simulink library "My_FI_Operations_ML2017a"  (R2017a)
settings: Solver=VariableStepAuto  StartTime=0.0  StopTime=10.0  RelTol=1e-3
settings Model: Creator=kolbe  LastModifiedBy=kolbe
settings DataIOCC: ReturnWorkspaceOutputs=on
settings SFSimCC: SimUseLocalCustomCode=on
settings RTWCC: RTWUseLocalCustomCode=on

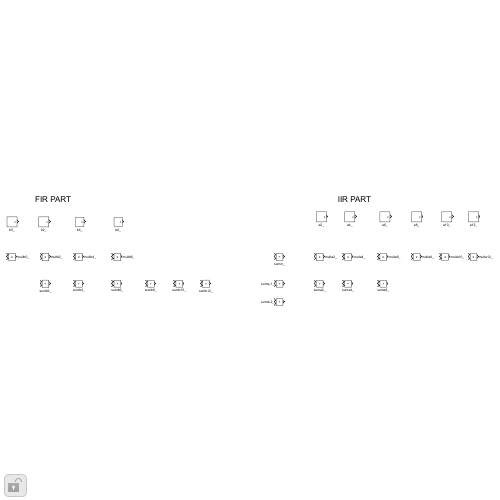
[thumbnail: Simulink's stored preview of the top-level diagram]
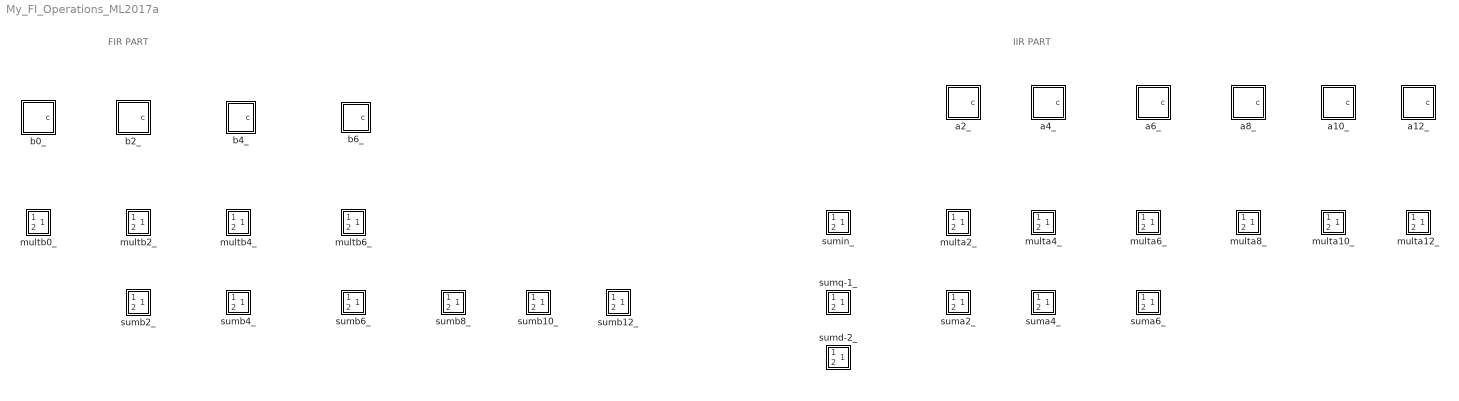
== system My_FI_Operations_ML2017a ==
  note: FIR PART
  note: IIR PART
  a10_ : Subsystem
  a12_ : Subsystem
  a2_ : Subsystem
  a4_ : Subsystem
  a6_ : Subsystem
  a8_ : Subsystem
  b0_ : Subsystem
  b2_ : Subsystem
  b4_ : Subsystem
  b6_ : Subsystem
  multa10_ : Subsystem
      mask Display: disp('x')
  multa12_ : Subsystem
      mask Display: disp('x')
  multa2_ : Subsystem
      mask Display: disp('x')
  multa4_ : Subsystem
      mask Display: disp('x')
  multa6_ : Subsystem
      mask Display: disp('x')
  multa8_ : Subsystem
      mask Display: disp('x')
  multb0_ : Subsystem
      mask Display: disp('x')
  multb2_ : Subsystem
      mask Display: disp('x')
  multb4_ : Subsystem
      mask Display: disp('x')
  multb6_ : Subsystem
      mask Display: disp('x')
  suma2_ : Subsystem
      mask Display: disp('+')
  suma4_ : Subsystem
      mask Display: disp('+')
  suma6_ : Subsystem
      mask Display: disp('+')
  sumb10_ : Subsystem
      mask Display: disp('+')
  sumb12_ : Subsystem
      mask Display: disp('+')
  sumb2_ : Subsystem
      mask Display: disp('+')
  sumb4_ : Subsystem
      mask Display: disp('+')
  sumb6_ : Subsystem
      mask Display: disp('+')
  sumb8_ : Subsystem
      mask Display: disp('+')
  sumd-2_ : Subsystem
      mask Display: disp('+')
  sumin_ : Subsystem
      mask Display: disp('+')
  sumq-1_ : Subsystem
      mask Display: disp('+')

== system My_FI_Operations_ML2017a/a10_ ==
  a10_ : Constant  Value=-1.218261718750000  OutDataTypeStr=fixdt(1,15,11)
  c : Outport
  wires:
  a10_/1 -> c/1

== system My_FI_Operations_ML2017a/a12_ ==
  a12_ : Constant  Value=-0.203125000000000  OutDataTypeStr=fixdt(1,15,11)
  c : Outport
  wires:
  a12_/1 -> c/1

== system My_FI_Operations_ML2017a/a2_ ==
  a2_ : Constant  Value=-3.291503906250000  OutDataTypeStr=fixdt(1,15,11)
  c : Outport
  wires:
  a2_/1 -> c/1

== system My_FI_Operations_ML2017a/a4_ ==
  a4_ : Constant  Value=-5.456054687500000  OutDataTypeStr=fixdt(1,15,11)
  c : Outport
  wires:
  a4_/1 -> c/1

== system My_FI_Operations_ML2017a/a6_ ==
  a6_ : Constant  Value=-5.414062500000000  OutDataTypeStr=fixdt(1,15,11)
  c : Outport
  wires:
  a6_/1 -> c/1

== system My_FI_Operations_ML2017a/a8_ ==
  a8_ : Constant  Value=-3.354492187500000  OutDataTypeStr=fixdt(1,15,11)
  c : Outport
  wires:
  a8_/1 -> c/1

== system My_FI_Operations_ML2017a/b0_ ==
  b0_ : Constant  Value=0.004394531250000  OutDataTypeStr=fixdt(1,12,11)
  c : Outport
  wires:
  b0_/1 -> c/1

== system My_FI_Operations_ML2017a/b2_ ==
  b2_ : Constant  Value=-0.010742187500000  OutDataTypeStr=fixdt(1,12,11)
  c : Outport
  wires:
  b2_/1 -> c/1

== system My_FI_Operations_ML2017a/b4_ ==
  b4_ : Constant  Value=0.018554687500000  OutDataTypeStr=fixdt(1,12,11)
  c : Outport
  wires:
  b4_/1 -> c/1

== system My_FI_Operations_ML2017a/b6_ ==
  b6_ : Constant  Value=-0.021484375000000  OutDataTypeStr=fixdt(1,12,11)
  c : Outport
  wires:
  b6_/1 -> c/1

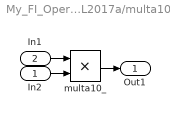
== system My_FI_Operations_ML2017a/multa10_ ==
  In2 : Inport
  In1 : Inport  Port=2
  multa10_ : Product  OutDataTypeStr=fixdt(1,26,24-10+FL)  RndMeth=Nearest  SaturateOnIntegerOverflow=on
  Out1 : Outport
  wires:
  In1/1 -> multa10_/1
  In2/1 -> multa10_/2
  multa10_/1 -> Out1/1

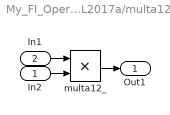
== system My_FI_Operations_ML2017a/multa12_ ==
  In2 : Inport
  In1 : Inport  Port=2
  multa12_ : Product  OutDataTypeStr=fixdt(1,27,26-10+FL)  RndMeth=Nearest  SaturateOnIntegerOverflow=on
  Out1 : Outport
  wires:
  In2/1 -> multa12_/2
  In1/1 -> multa12_/1
  multa12_/1 -> Out1/1

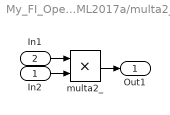
== system My_FI_Operations_ML2017a/multa2_ ==
  In2 : Inport
  In1 : Inport  Port=2
  multa2_ : Product  OutDataTypeStr=fixdt(1,39,36-10+FL)  RndMeth=Nearest  SaturateOnIntegerOverflow=on
  Out1 : Outport
  wires:
  In2/1 -> multa2_/2
  In1/1 -> multa2_/1
  multa2_/1 -> Out1/1

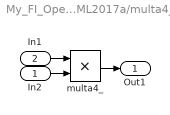
== system My_FI_Operations_ML2017a/multa4_ ==
  In2 : Inport
  In1 : Inport  Port=2
  multa4_ : Product  OutDataTypeStr=fixdt(1,44,40-10+FL)  RndMeth=Nearest  SaturateOnIntegerOverflow=on
  Out1 : Outport
  wires:
  In1/1 -> multa4_/1
  multa4_/1 -> Out1/1
  In2/1 -> multa4_/2

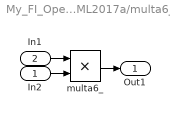
== system My_FI_Operations_ML2017a/multa6_ ==
  In2 : Inport
  In1 : Inport  Port=2
  multa6_ : Product  OutDataTypeStr=fixdt(1,29,25-10+FL)  RndMeth=Nearest  SaturateOnIntegerOverflow=on
  Out1 : Outport
  wires:
  In1/1 -> multa6_/1
  In2/1 -> multa6_/2
  multa6_/1 -> Out1/1

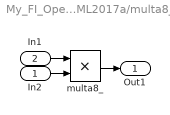
== system My_FI_Operations_ML2017a/multa8_ ==
  In2 : Inport
  In1 : Inport  Port=2
  multa8_ : Product  OutDataTypeStr=fixdt(1,36,33-10+FL)  RndMeth=Nearest  SaturateOnIntegerOverflow=on
  Out1 : Outport
  wires:
  In1/1 -> multa8_/1
  In2/1 -> multa8_/2
  multa8_/1 -> Out1/1

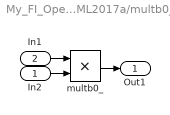
== system My_FI_Operations_ML2017a/multb0_ ==
  In2 : Inport
  In1 : Inport  Port=2
  multb0_ : Product  OutDataTypeStr=fixdt(1,22,21-10+FL)  RndMeth=Nearest  SaturateOnIntegerOverflow=on
  Out1 : Outport
  wires:
  In1/1 -> multb0_/1
  multb0_/1 -> Out1/1
  In2/1 -> multb0_/2

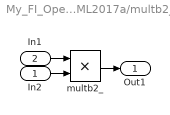
== system My_FI_Operations_ML2017a/multb2_ ==
  In2 : Inport
  In1 : Inport  Port=2
  multb2_ : Product  OutDataTypeStr=fixdt(1,21,20-10+FL)  RndMeth=Nearest  SaturateOnIntegerOverflow=on
  Out1 : Outport
  wires:
  multb2_/1 -> Out1/1
  In2/1 -> multb2_/2
  In1/1 -> multb2_/1

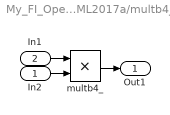
== system My_FI_Operations_ML2017a/multb4_ ==
  In2 : Inport
  In1 : Inport  Port=2
  multb4_ : Product  OutDataTypeStr=fixdt(1,21,20-10+FL)  RndMeth=Nearest  SaturateOnIntegerOverflow=on
  Out1 : Outport
  wires:
  multb4_/1 -> Out1/1
  In1/1 -> multb4_/1
  In2/1 -> multb4_/2

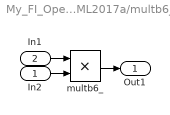
== system My_FI_Operations_ML2017a/multb6_ ==
  In2 : Inport
  In1 : Inport  Port=2
  multb6_ : Product  OutDataTypeStr=fixdt(1,20,19-10+FL)  RndMeth=Nearest  SaturateOnIntegerOverflow=on
  Out1 : Outport
  wires:
  In1/1 -> multb6_/1
  multb6_/1 -> Out1/1
  In2/1 -> multb6_/2

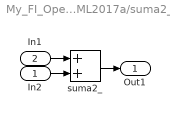
== system My_FI_Operations_ML2017a/suma2_ ==
  In2 : Inport
  In1 : Inport  Port=2
  suma2_ : Sum  OutDataTypeStr=fixdt(1,33,29-10+FL)  RndMeth=Nearest  SaturateOnIntegerOverflow=on
  Out1 : Outport
  wires:
  In2/1 -> suma2_/2
  suma2_/1 -> Out1/1
  In1/1 -> suma2_/1

== system My_FI_Operations_ML2017a/suma4_ ==
  In1 : Inport
  In2 : Inport  Port=2
  suma4_ : Sum  OutDataTypeStr=fixdt(1,42,38-10+FL)  RndMeth=Nearest  SaturateOnIntegerOverflow=on
  Out1 : Outport
  wires:
  suma4_/1 -> Out1/1
  In2/1 -> suma4_/2
  In1/1 -> suma4_/1

== system My_FI_Operations_ML2017a/suma6_ ==
  In1 : Inport
  In2 : Inport  Port=2
  suma6_ : Sum  OutDataTypeStr=fixdt(1,28,24-10+FL)  RndMeth=Nearest  SaturateOnIntegerOverflow=on
  Out1 : Outport
  wires:
  In1/1 -> suma6_/1
  In2/1 -> suma6_/2
  suma6_/1 -> Out1/1

== system My_FI_Operations_ML2017a/sumb10_ ==
  In2 : Inport
  In1 : Inport  Port=2
  sumb10_ : Sum  OutDataTypeStr=fixdt(1,22,21-10+FL)  RndMeth=Nearest  SaturateOnIntegerOverflow=on
  Out1 : Outport
  wires:
  In1/1 -> sumb10_/1
  In2/1 -> sumb10_/2
  sumb10_/1 -> Out1/1

== system My_FI_Operations_ML2017a/sumb12_ ==
  In2 : Inport
  In1 : Inport  Port=2
  sumb12_ : Sum  OutDataTypeStr=fixdt(1,22,21-10+FL)  RndMeth=Nearest  SaturateOnIntegerOverflow=on
  Out1 : Outport
  wires:
  In1/1 -> sumb12_/1
  sumb12_/1 -> Out1/1
  In2/1 -> sumb12_/2

== system My_FI_Operations_ML2017a/sumb2_ ==
  In2 : Inport
  In1 : Inport  Port=2
  sumb2_ : Sum  OutDataTypeStr=fixdt(1,22,21-10+FL)  RndMeth=Nearest  SaturateOnIntegerOverflow=on
  Out1 : Outport
  wires:
  In1/1 -> sumb2_/1
  In2/1 -> sumb2_/2
  sumb2_/1 -> Out1/1

== system My_FI_Operations_ML2017a/sumb4_ ==
  In2 : Inport
  In1 : Inport  Port=2
  sumb4_ : Sum  OutDataTypeStr=fixdt(1,22,21-10+FL)  RndMeth=Nearest  SaturateOnIntegerOverflow=on
  Out1 : Outport
  wires:
  In1/1 -> sumb4_/1
  In2/1 -> sumb4_/2
  sumb4_/1 -> Out1/1

== system My_FI_Operations_ML2017a/sumb6_ ==
  In2 : Inport
  In1 : Inport  Port=2
  sumb6_ : Sum  OutDataTypeStr=fixdt(1,22,21-10+FL)  RndMeth=Nearest  SaturateOnIntegerOverflow=on
  Out1 : Outport
  wires:
  sumb6_/1 -> Out1/1
  In1/1 -> sumb6_/1
  In2/1 -> sumb6_/2

== system My_FI_Operations_ML2017a/sumb8_ ==
  In2 : Inport
  In1 : Inport  Port=2
  sumb8_ : Sum  OutDataTypeStr=fixdt(1,22,21-10+FL)  RndMeth=Nearest  SaturateOnIntegerOverflow=on
  Out1 : Outport
  wires:
  sumb8_/1 -> Out1/1
  In1/1 -> sumb8_/1
  In2/1 -> sumb8_/2

== system My_FI_Operations_ML2017a/sumd-2_ ==
  In1 : Inport
  In2 : Inport  Port=2
  sumd-2_ : Sum  OutDataTypeStr=fixdt(1,34,30-10+FL)  RndMeth=Nearest
  Out1 : Outport
  wires:
  In2/1 -> sumd-2_/2
  sumd-2_/1 -> Out1/1
  In1/1 -> sumd-2_/1

== system My_FI_Operations_ML2017a/sumin_ ==
  In1 : Inport
  In2 : Inport  Port=2
  sumin_ : Sum  OutDataTypeStr=fixdt(1,36,34-10+FL)  RndMeth=Nearest  SaturateOnIntegerOverflow=on
  Out1 : Outport
  wires:
  In2/1 -> sumin_/2
  In1/1 -> sumin_/1
  sumin_/1 -> Out1/1

== system My_FI_Operations_ML2017a/sumq-1_ ==
  In2 : Inport
  In1 : Inport  Port=2
  sumq-1_ : Sum  OutDataTypeStr=fixdt(1,39,35-10+FL)  RndMeth=Nearest  SaturateOnIntegerOverflow=on
  Out1 : Outport
  wires:
  sumq-1_/1 -> Out1/1
  In2/1 -> sumq-1_/2
  In1/1 -> sumq-1_/1
